simulink model "PC3_ex1"  (R2016b)
settings: Solver=VariableStepAuto  StartTime=0.0  StopTime=10.0  MaxStep=0.01  RelTol=1e-3
values from neighbouring files (symbols this model uses):
  dx0 = randn()    [PC3_ex1.m]
  K1 = lqr(A, B, R, Q1)    [PC3_ex1.m]
  K2 = lqr(A, B, R, Q2)    [PC3_ex1.m]
  K3 = lqr(A, B, R, Q3)    [PC3_ex1.m]
  x0 = randn()    [PC3_ex1.m]
settings Model: Creator=BOUDOT  LastModifiedBy=BOUDOT

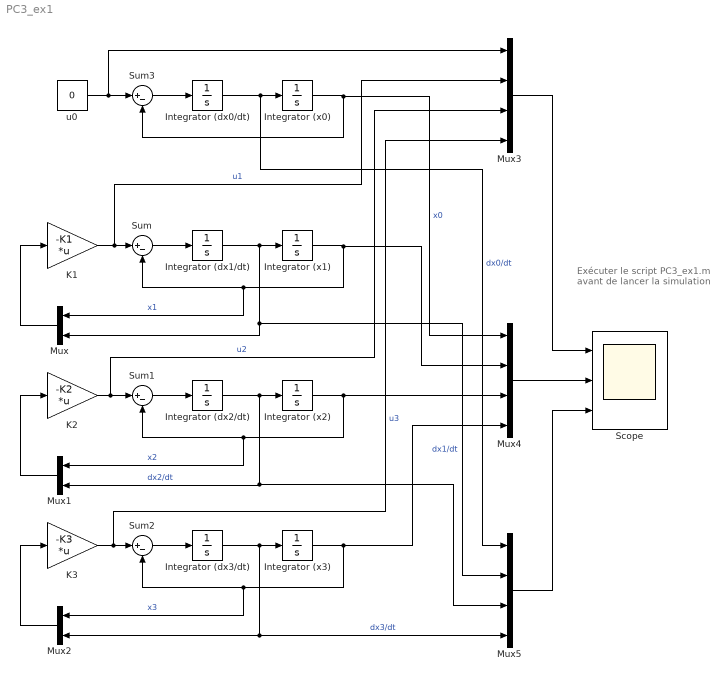
== system PC3_ex1 ==
  note: Exécuter le script PC3_ex1.m avant de lancer la simulation
  Integrator (dx0/dt) : Integrator  InitialCondition=dx0
  Integrator (dx1/dt) : Integrator  InitialCondition=dx0
  Integrator (dx2/dt) : Integrator  InitialCondition=dx0
  Integrator (dx3/dt) : Integrator  InitialCondition=dx0
  Integrator (x0) : Integrator  InitialCondition=x0
  Integrator (x1) : Integrator  InitialCondition=x0
  Integrator (x2) : Integrator  InitialCondition=x0
  Integrator (x3) : Integrator  InitialCondition=x0
  "K1 " : Gain  Gain=-K1  Multiplication=Matrix(K*u)
  K2 : Gain  Gain=-K2  Multiplication=Matrix(K*u)
  K3 : Gain  Gain=-K3  Multiplication=Matrix(K*u)
  Mux : Mux  Inputs=2
  Mux1 : Mux  Inputs=2
  Mux2 : Mux  Inputs=2
  Mux3 : Mux
  Mux4 : Mux
  Mux5 : Mux
  Scope : Scope  NumInputPorts=3
  Sum{,1..3} (4 alike) : Sum  Inputs=|+-
  u0 : Constant  Value=0
  wires:
  Integrator (dx1/dt)/1 -> Mux/2, Mux5/2, Integrator (x1)/1  "dx1/dt"
  Sum/1 -> Integrator (dx1/dt)/1
  Integrator (x1)/1 -> Mux4/2, Sum/2, Mux/1  "x1"
  "K1 "/1 -> Mux3/2, Sum/1  "u1"
  Mux/1 -> "K1 "/1
  Integrator (dx2/dt)/1 -> Integrator (x2)/1, Mux5/3, Mux1/2  "dx2/dt"
  Sum1/1 -> Integrator (dx2/dt)/1
  Integrator (x2)/1 -> Mux4/3, Mux1/1, Sum1/2  "x2"
  K2/1 -> Mux3/3, Sum1/1  "u2"
  Mux1/1 -> K2/1
  Integrator (dx3/dt)/1 -> Mux5/4, Mux2/2, Integrator (x3)/1  "dx3/dt"
  Sum2/1 -> Integrator (dx3/dt)/1
  Integrator (x3)/1 -> Mux4/4, Sum2/2, Mux2/1  "x3"
  K3/1 -> Mux3/4, Sum2/1  "u3"
  Mux2/1 -> K3/1
  Integrator (dx0/dt)/1 -> Mux5/1, Integrator (x0)/1  "dx0/dt"
  Sum3/1 -> Integrator (dx0/dt)/1
  Integrator (x0)/1 -> Mux4/1, Sum3/2  "x0"
  u0/1 -> Mux3/1, Sum3/1
  Mux4/1 -> Scope/2
  Mux3/1 -> Scope/1
  Mux5/1 -> Scope/3
